simulink model "matlabfuction"  (R2018a)
settings: Solver=FixedStepAuto  StartTime=0.0  StopTime=1e-3  FixedStep=1e-6  RelTol=1e-3
settings Model: Creator=user  LastModifiedBy=user

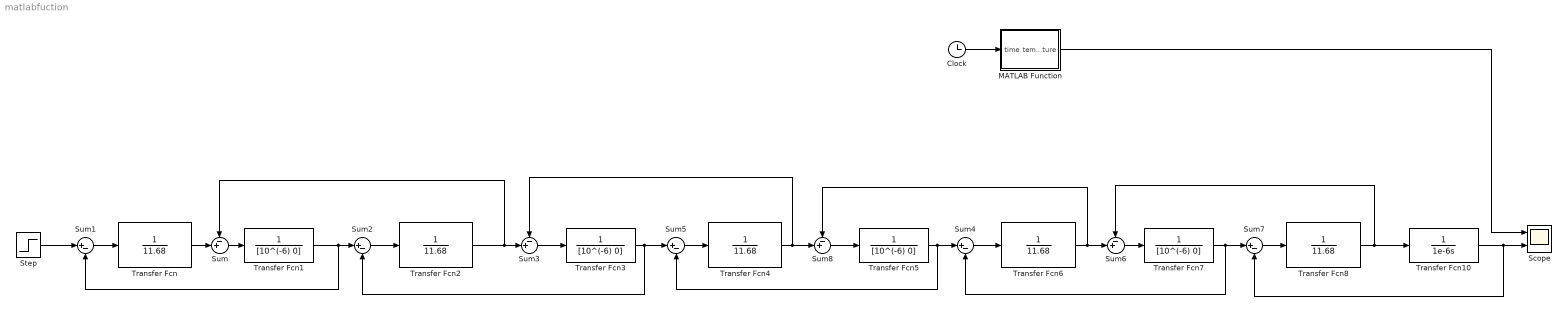
== system matlabfuction ==
  Clock : Clock
  MATLAB Function : MATLAB Function  TreatAsAtomicUnit=on
  Scope : Scope  NumInputPorts=2
  Step : Step  SampleTime=0
  Sum{,3,6,8} (4 alike) : Sum  Inputs=-+|
  Sum{1..2,4..5,7} (5 alike) : Sum  Inputs=|+-
  Transfer Fcn{,2,4,6,8} (5 alike) : TransferFcn  Denominator=[11.68]
  Transfer Fcn{1,3,5,7} (4 alike) : TransferFcn  Denominator=[10^(-6) 0]
  Transfer Fcn10 : TransferFcn  Denominator=[1e-6 0]
  wires:
  Sum1/1 -> Transfer Fcn/1
  Transfer Fcn1/1 -> Sum2/1, Sum1/2
  Step/1 -> Sum1/1
  Transfer Fcn/1 -> Sum/2
  Sum/1 -> Transfer Fcn1/1
  Sum2/1 -> Transfer Fcn2/1
  Transfer Fcn2/1 -> Sum3/2, Sum/1
  Transfer Fcn3/1 -> Sum5/1, Sum2/2
  Sum3/1 -> Transfer Fcn3/1
  Transfer Fcn5/1 -> Sum4/1, Sum5/2
  Sum5/1 -> Transfer Fcn4/1
  Sum7/1 -> Transfer Fcn8/1
  Transfer Fcn7/1 -> Sum7/1, Sum4/2
  Sum6/1 -> Transfer Fcn7/1
  Transfer Fcn8/1 -> Transfer Fcn10/1, Sum6/1
  Sum4/1 -> Transfer Fcn6/1
  Sum8/1 -> Transfer Fcn5/1
  Transfer Fcn6/1 -> Sum6/2, Sum8/1
  Transfer Fcn4/1 -> Sum8/2, Sum3/1
  Transfer Fcn10/1 -> Scope/2, Sum7/2
  Clock/1 -> MATLAB Function/1(time)
  MATLAB Function/1(temperature) -> Scope/1

== matlab function matlabfuction/MATLAB Function ==
  data: time input; temperature output
function temperature = calculateTemp(time)
L=5;
rho=2.70;
k=0.497;
c=0.215;

alpha=k/(rho*c);
scale=1e5;
if(time>0)
    temperature=erfc( L./(2*sqrt(alpha*time*scale)));
else
    temperature = time;
end
end
